simulink model "lab3_step8"  (R2019b)
settings: Solver=VariableStepAuto  StartTime=0.0  StopTime=stop_time  RelTol=1e-3
InitFcn:
  | sm_callback_init
StopFcn:
  | sm_callback_stop
values from neighbouring files (symbols this model uses):
  mp = sm_init_avalon_signals(mp)    [sm_callback_init.m]    (also in sm_callback_stop.m = sm_stop_verify(mp))
libraries: simulink x2
settings Model: Creator=yassi  LastModifiedBy=yassi
settings DataIOCC: ReturnWorkspaceOutputs=off

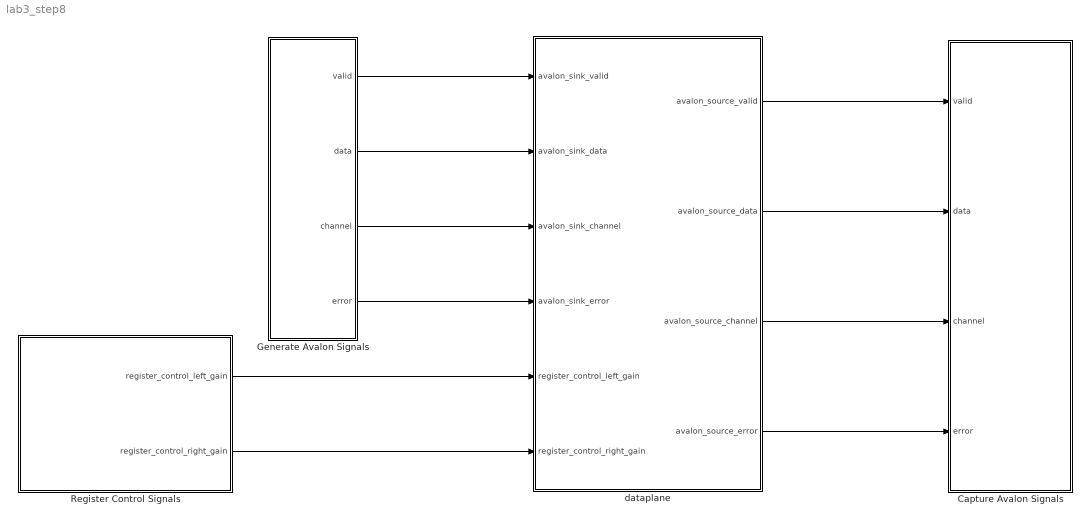
== system lab3_step8 ==
  Capture Avalon Signals : Subsystem
  Generate Avalon Signals : Subsystem
  Register Control Signals : Subsystem
  dataplane : Subsystem
  wires:
  Generate Avalon Signals/1(valid) -> dataplane/1(avalon_sink_valid)
  Generate Avalon Signals/2(data) -> dataplane/2(avalon_sink_data)
  Generate Avalon Signals/3(channel) -> dataplane/3(avalon_sink_channel)
  Generate Avalon Signals/4(error) -> dataplane/4(avalon_sink_error)
  dataplane/1(avalon_source_valid) -> Capture Avalon Signals/1(valid)
  dataplane/2(avalon_source_data) -> Capture Avalon Signals/2(data)
  dataplane/3(avalon_source_channel) -> Capture Avalon Signals/3(channel)
  dataplane/4(avalon_source_error) -> Capture Avalon Signals/4(error)
  Register Control Signals/1(register_control_left_gain) -> dataplane/5(register_control_left_gain)
  Register Control Signals/2(register_control_right_gain) -> dataplane/6(register_control_right_gain)

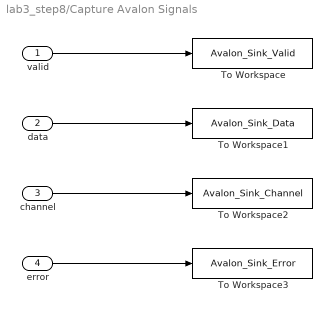
== system lab3_step8/Capture Avalon Signals ==
  valid : Inport
  data : Inport  Port=2
  channel : Inport  Port=3
  error : Inport  Port=4
  To Workspace : ToWorkspace  VariableName=Avalon_Sink_Valid  SaveFormat=Timeseries  SampleTime=-1
  To Workspace1 : ToWorkspace  VariableName=Avalon_Sink_Data  SaveFormat=Timeseries  SampleTime=-1
  To Workspace2 : ToWorkspace  VariableName=Avalon_Sink_Channel  SaveFormat=Timeseries  SampleTime=-1
  To Workspace3 : ToWorkspace  VariableName=Avalon_Sink_Error  SaveFormat=Timeseries  SampleTime=-1
  wires:
  valid/1 -> To Workspace/1
  data/1 -> To Workspace1/1
  channel/1 -> To Workspace2/1
  error/1 -> To Workspace3/1

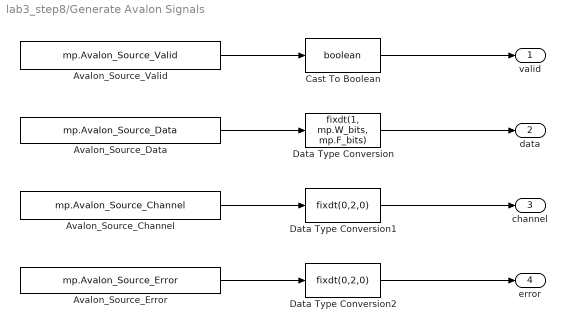
== system lab3_step8/Generate Avalon Signals ==
  Avalon_Source_Channel : FromWorkspace  VariableName=mp.Avalon_Source_Channel  OutDataTypeStr=double  SampleTime=mp.Ts_system
  Avalon_Source_Data : FromWorkspace  VariableName=mp.Avalon_Source_Data  OutDataTypeStr=double  SampleTime=mp.Ts_system
  Avalon_Source_Error : FromWorkspace  VariableName=mp.Avalon_Source_Error  OutDataTypeStr=double  SampleTime=mp.Ts_system
  Avalon_Source_Valid : FromWorkspace  VariableName=mp.Avalon_Source_Valid  OutDataTypeStr=double  SampleTime=mp.Ts_system
  Cast To Boolean : DataTypeConversion  OutDataTypeStr=boolean
  Data Type Conversion : DataTypeConversion  OutDataTypeStr=fixdt(1, mp.W_bits, mp.F_bits)
  Data Type Conversion1 : DataTypeConversion  OutDataTypeStr=fixdt(0,2,0)
  Data Type Conversion2 : DataTypeConversion  OutDataTypeStr=fixdt(0,2,0)
  valid : Outport
  data : Outport  Port=2
  channel : Outport  Port=3
  error : Outport  Port=4
  wires:
  Avalon_Source_Valid/1 -> Cast To Boolean/1
  Avalon_Source_Data/1 -> Data Type Conversion/1
  Avalon_Source_Channel/1 -> Data Type Conversion1/1
  Avalon_Source_Error/1 -> Data Type Conversion2/1
  Cast To Boolean/1 -> valid/1
  Data Type Conversion/1 -> data/1
  Data Type Conversion1/1 -> channel/1
  Data Type Conversion2/1 -> error/1

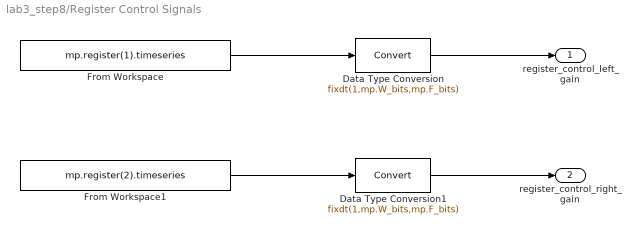
== system lab3_step8/Register Control Signals ==
  Data Type Conversion : DataTypeConversion  OutDataTypeStr=fixdt(1,mp.W_bits,mp.F_bits)
  Data Type Conversion1 : DataTypeConversion  OutDataTypeStr=fixdt(1,mp.W_bits,mp.F_bits)
  From Workspace : FromWorkspace  VariableName=mp.register(1).timeseries  OutDataTypeStr=double  SampleTime=mp.Ts_system
  From Workspace1 : FromWorkspace  VariableName=mp.register(2).timeseries  OutDataTypeStr=double  SampleTime=mp.Ts_system
  register_control_left_gain : Outport
  register_control_right_gain : Outport  Port=2
  wires:
  Data Type Conversion1/1 -> register_control_right_gain/1
  Data Type Conversion/1 -> register_control_left_gain/1
  From Workspace/1 -> Data Type Conversion/1
  From Workspace1/1 -> Data Type Conversion1/1

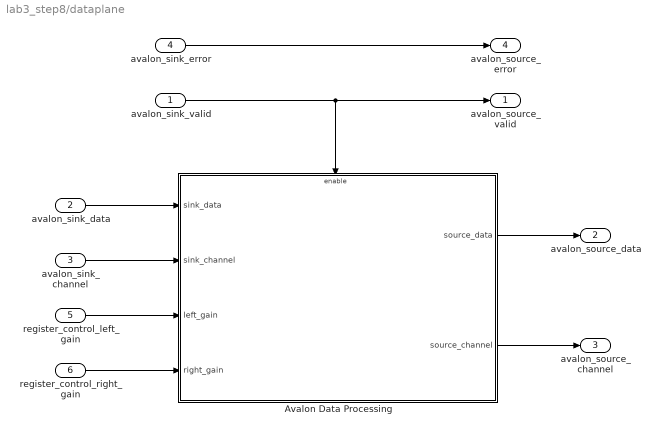
== system lab3_step8/dataplane ==
  avalon_sink_valid : Inport
  avalon_sink_data : Inport  Port=2
  avalon_sink_channel : Inport  Port=3
  avalon_sink_error : Inport  Port=4
  register_control_left_gain : Inport  Port=5
  register_control_right_gain : Inport  Port=6
  Avalon Data Processing : Subsystem  TreatAsAtomicUnit=on
  avalon_source_valid : Outport
  avalon_source_data : Outport  Port=2
  avalon_source_channel : Outport  Port=3
  avalon_source_error : Outport  Port=4
  wires:
  avalon_sink_error/1 -> avalon_source_error/1
  avalon_sink_valid/1 -> avalon_source_valid/1, Avalon Data Processing/Enable
  avalon_sink_data/1 -> Avalon Data Processing/1(sink_data)
  avalon_sink_channel/1 -> Avalon Data Processing/2(sink_channel)
  register_control_left_gain/1 -> Avalon Data Processing/3(left_gain)
  register_control_right_gain/1 -> Avalon Data Processing/4(right_gain)
  Avalon Data Processing/1(source_data) -> avalon_source_data/1
  Avalon Data Processing/2(source_channel) -> avalon_source_channel/1

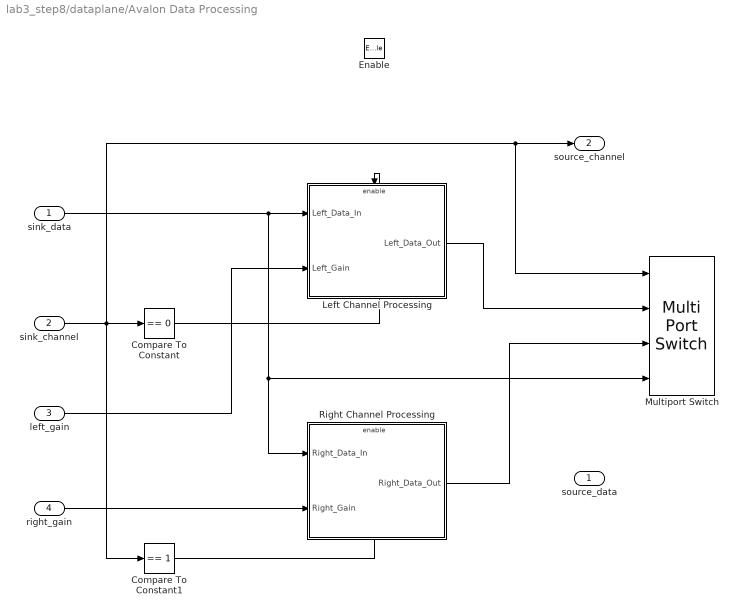
== system lab3_step8/dataplane/Avalon Data Processing ==
  sink_data : Inport
  sink_channel : Inport  Port=2
  left_gain : Inport  Port=3
  right_gain : Inport  Port=4
  Enable : EnablePort
  Compare To Constant : simulink/Logic and Bit Operations/Compare To Constant  relop===  const=0  OutDataTypeStr=boolean
  Compare To Constant1 : simulink/Logic and Bit Operations/Compare To Constant  relop===  const=1  OutDataTypeStr=boolean
  Left Channel Processing : Subsystem  TreatAsAtomicUnit=on
  Multiport Switch : MultiPortSwitch  DataPortOrder=Zero-based contiguous  zeroidx=on
  Right Channel Processing : Subsystem  TreatAsAtomicUnit=on
  source_data : Outport
  source_channel : Outport  Port=2
  wires:
  sink_data/1 -> Right Channel Processing/1(Right_Data_In), Multiport Switch/4, Left Channel Processing/1(Left_Data_In)
  sink_channel/1 -> Multiport Switch/1, source_channel/1, Compare To Constant1/1, Compare To Constant/1
  Compare To Constant/1 -> Left Channel Processing/Enable
  Compare To Constant1/1 -> Right Channel Processing/Enable
  left_gain/1 -> Left Channel Processing/2(Left_Gain)
  right_gain/1 -> Right Channel Processing/2(Right_Gain)
  Left Channel Processing/1(Left_Data_Out) -> Multiport Switch/2
  Right Channel Processing/1(Right_Data_Out) -> Multiport Switch/3

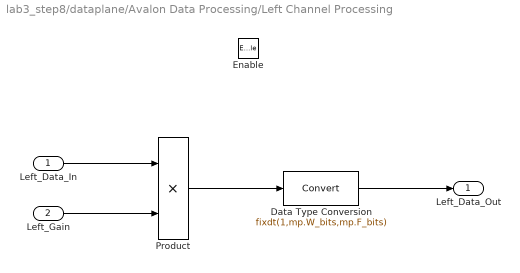
== system lab3_step8/dataplane/Avalon Data Processing/Left Channel Processing ==
  Left_Data_In : Inport
  Left_Gain : Inport  Port=2
  Enable : EnablePort
  Data Type Conversion : DataTypeConversion  OutDataTypeStr=fixdt(1,mp.W_bits,mp.F_bits)
  Product : Product
  Left_Data_Out : Outport
  wires:
  Data Type Conversion/1 -> Left_Data_Out/1
  Product/1 -> Data Type Conversion/1
  Left_Data_In/1 -> Product/1
  Left_Gain/1 -> Product/2

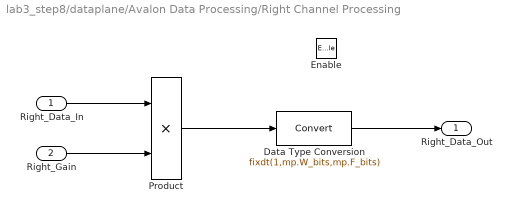
== system lab3_step8/dataplane/Avalon Data Processing/Right Channel Processing ==
  Right_Data_In : Inport
  Right_Gain : Inport  Port=2
  Enable : EnablePort
  Data Type Conversion : DataTypeConversion  OutDataTypeStr=fixdt(1,mp.W_bits,mp.F_bits)
  Product : Product
  Right_Data_Out : Outport
  wires:
  Data Type Conversion/1 -> Right_Data_Out/1
  Product/1 -> Data Type Conversion/1
  Right_Data_In/1 -> Product/1
  Right_Gain/1 -> Product/2
